simulink model "MenakaModel"  (R2022a)
settings: Solver=ode23tb  StartTime=0.0  StopTime=4  MaxStep=10/(60*24)  RelTol=1e-3
model workspace (MAT data in the model file):
  clima__A_c = 3295.16408265
  clima__A_f = 3100.53942116
  clima__G0 = [0.05; 0.00070738]
  clima__H = 7.9995824611
  clima__T0 = [287.15; 287.15; 287.15; 287.15]
  clima__T_ss = 280.150340169
  clima__alpha_c = 0.0100640347387
  clima__alpha_f = 0.0111385012129
  clima__alpha_i = 0.1
  clima__c_s = [1081 1081]
  clima__cd_c = 8736
  clima__d_c = 1.5
  clima__hour0 = 1
  clima__int_air_speed = 0.5
  clima__l_s = [0.1 0.1]
  clima__lam_s = [2.5 0.85]
  clima__minWindows = 0.299965865643
  clima__rhod_s = [2600 2500]
  clima__tau_c = 1
  crop__A_v = 2080
  crop__C = [0.01 0.001 0.01 0.01]
  crop__C_buf_max = 0.02
  crop__C_wv = 0.2
  crop__Chi_nutrients = [0.015625; 0.0104166666667; 0.00520833333333; 0.00208333333333; 0.00208333333333; 0.00104166666667; 0; 0]
  crop__N = [0; 0; 0; 0; 0; 0; 0; 0]
  crop__R = [0 0 0]
  crop__T_max_v = 40
  crop__T_max_v24 = 27
  crop__T_min_v = 6
  crop__T_min_v24 = 14
  crop__T_sum_end = 1035
  crop__T_v_start_fruit = 1100
  crop__Tsum = 0
  crop__Tv = 288
  crop__b_N_uptake = 0.5
  crop__c_fruit_g = 0.27
  crop__c_fruit_m = 2.3e-07
  crop__c_leaf_g = 0.28
  crop__c_leaf_m = 3.47e-07
  crop__c_stem_g = 0.3
  crop__c_stem_m = 1.47e-07
  crop__fraction_DM = 0.08
  crop__int_air_speed = 0.5
  crop__min_water_capacity = 0.1
  crop__plants_density = 2.1562
  crop__rg_fruit = 2e-07
  crop__rg_leaf = 9.5e-08
  crop__rg_stem = 7.4e-08
  crop__s_buforg_buf = -5000
  crop__s_max_T = 0.5793
  crop__s_max_T24 = 1.3904
  crop__s_min_T = -0.869
  crop__s_min_T24 = -1.1587
  heater__A_e = 0.0001
  heater__A_i = 0.008
  heater__T = 288
  heater__c = 5e-10
  heater__power = 60000000
  screen__Power = 100
  screen__Radthreshold = 900
  screen__beta = 2.23564167038e-14
  screen__gamma_max = 2.26308905438e-14
  screen__velocity = 0.333333333333
  subtrate__C_ws = 0.1
  subtrate__N = [0; 0; 0; 0; 0; 0; 0; 0]
  subtrate__Nmin_subs = 1e-09
  subtrate__Vmax_subs = 10
  subtrate__Vmin_subs = 0.01
  subtrate__sigma_max = 1
  subtrate__sigma_min = 1
  tomato__Cfruit0 = 0.001
  windows__AR = 19.9974923936
  windows__Power = 100
  windows__RadThreshold = 10
  windows__max_night = 10
  windows__tau = 600
undefined symbols (not defined in the file or in its folder): CO2_ppm_ext, Gain_control_Tv_mean, Gain_control_Tv_mean_superior, gain_max_night, GAIN_WIN, Hmax, Hstart, max_night, maxvelocity, RadTh_windows, Radthhold, shift_temp_heat, tau_win, tend_crop1, tend_crop2, tinit_crop1, tinit_crop2, Tmax, Tmax_mean, Tstart, Tven_max, Tven_start, WinAR
libraries: HORTISIM x26, simulink x6
(part 2 of 5)

== system MenakaModel/Control System/Control System Proportional (Ti) + Tmu Windows Relay/Subsystem1 ==
  " " : Inport
  Bus Creator1 : BusCreator  Inputs=2
  Bus Selector : BusSelector  OutputSignals=value,AR
  Rate Limiter : RateLimiter  RisingSlewLimit=maxvelocity*60*24  FallingSlewLimit=-maxvelocity*60*24  SampleTimeMode=inherited
  Out1 : Outport
  wires:
  " "/1 -> Bus Selector/1
  Bus Selector/2 -> Bus Creator1/2  "<AR>"
  Bus Selector/1 -> Rate Limiter/1  "<value>"
  Bus Creator1/1 -> Out1/1
  Rate Limiter/1 -> Bus Creator1/1  "value"

== system MenakaModel/Control System/Control System Proportional (Ti) + Tmu Windows Relay/Windows Controler ==
  note: Subsystem1
  In Bus Element1 : Inport  PortName=IC  Element=Temp.Tair
  In Bus Element2 : Inport  PortName=IC  Element=Gas.HRInt
  Tstart : Inport  Port=2
  Tmax : Inport  Port=3
  Hstart : Inport  Port=4
  Hmax : Inport  Port=5
  R : Inport  Port=6
  Abs : Abs  ZeroCross=off  SaturateOnIntegerOverflow=off
  Bus Creator : BusCreator  Inputs=2
  Bus Selector : BusSelector  OutputSignals=Rad
  Constant : Constant  Value=AR
  Gain : Gain  Gain=100/tau
  Gain1 : Gain  Gain=Power
  Gain2 : Gain  Gain=24*3600*GAIN_WIN
  Integrator : Integrator
  Integrator1 : Integrator  InitialConditionSource=external
  Minus : Sum  Inputs=+-
  Minus1 : Sum  Inputs=+-
  Sec2Days : Gain  Gain=24*3600
  Subsystem : Subsystem
      settings: PortSchema="{\"entries\":[{\"content\":{\"sides\":[{\"content\":{\"connectorIds\":[\"In1\",\"In2\",\"In3\",\"In4\",\"In5\",\"In6\"]},\"type\":\"ConnectorPlacement.EquallySpacedRectSide\",\"uuid\":\"18d05740-181f-409c-94ea-b42b6e57ea74\"},{\"content\":{\"connectorIds\":[\"Out1\"],\"side\":\"RIGHT\"},\"type\":\"ConnectorPlacement.EquallySpacedRectSide\",\"uuid\":\"978406c3-d241-44cd-a3e7-fe734e3a171e\"},{\"content\":{\"connectorIds\":[\"In7\"],\"side\":\"TOP\"},\"type\":\"ConnectorPlacement.EquallySpacedRectSide\",\"uuid\":\"b3c10a0e-c6d9-4444-97f2-9f0c7dea8ec9\"}]},\"type\":\"ConnectorPlacement.EquallySpacedConnector\",\"uuid\":\"429bf3f5-5806-495e-b66b-96810540e6d1\"}],\"packageUris\":[\"http://schema.mathworks.com/mf0/Connector/R2020b\"],\"version\":\"1.0\"}"
  Tanh : Trigonometry  Operator=tanh
  Windows : Outport
  Consumptions : Outport  Port=2
  tag scope: Rad_win=global
  wires:
  Tstart/1 -> Subsystem/1(Tstart)
  In Bus Element1/1 -> Subsystem/2(Ti)
  Tmax/1 -> Subsystem/3(Tmax)
  Integrator/1 -> Bus Creator/1, Minus/2  "value"
  In Bus Element2/1 -> Subsystem/4(HRInt)
  Hstart/1 -> Subsystem/5(HRStart)
  Hmax/1 -> Subsystem/6(HRMax)
  Subsystem/1(y) -> Minus/1
  Sec2Days/1 -> Integrator/1
  Gain1/1 -> Consumptions/1  "Power"
  Abs/1 -> Gain1/1
  Gain/1 -> Abs/1, Sec2Days/1
  Tanh/1 -> Gain/1
  Minus/1 -> Tanh/1
  Bus Creator/1 -> Windows/1
  Constant/1 -> Bus Creator/2  "AR"
  Gain2/1 -> Integrator1/1
  Minus1/1 -> Gain2/1
  Integrator1/1 -> [Rad_win], Subsystem/7(Rad), Minus1/2
  R/1 -> Bus Selector/1
  Bus Selector/1 -> Integrator1/2, Minus1/1  "<Rad>"

== system MenakaModel/Control System/ON//OFF - constant setpoints/Subsystem ==
  Heater : Inport
  C1 : Inport  Port=2
  C2 : Inport  Port=3
  Bus Selector : BusSelector  OutputSignals=HeatVars.QV,HeatVars.QT,A_v,CC
  Bus Selector1 : BusSelector  OutputSignals=HeatVars.QV,HeatVars.QT,CC
  "Scalar2Bus " : Subsystem
  Sum : Sum  Inputs=+++
  Sum1 : Sum  Inputs=++|
  Sum2 : Sum  Inputs=++|
  CoCl : Outport
  wires:
  C1/1 -> Bus Selector/1
  C2/1 -> Bus Selector1/1
  Bus Selector/4 -> Sum2/2  "<CC>"
  Sum/1 -> "Scalar2Bus "/1(QV)
  Sum1/1 -> "Scalar2Bus "/2(QT)
  Bus Selector/1 -> Sum/3  "<QV>"
  Bus Selector1/1 -> Sum/1  "<QV>"
  Bus Selector1/2 -> Sum1/1  "<QT>"
  Bus Selector/3 -> "Scalar2Bus "/3(A)  "<A_v>"
  "Scalar2Bus "/1(CoCl) -> CoCl/1
  Sum2/1 -> "Scalar2Bus "/4(CC)
  Bus Selector1/3 -> Sum2/1  "<CC>"
  Heater/1 -> Sum/2
  Bus Selector/2 -> Sum1/2  "<QT>"

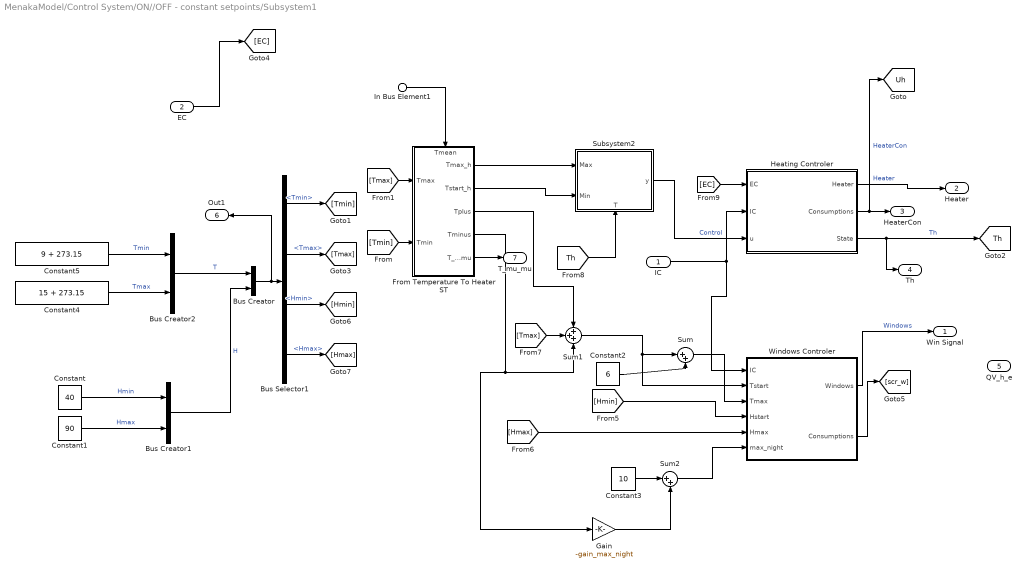
== system MenakaModel/Control System/ON//OFF - constant setpoints/Subsystem1 ==
  IC : Inport
  EC : Inport  Port=2
  In Bus Element1 : Inport  Port=3  PortName=Crop  Element=HeatVars.TvegMean
  Bus Creator : BusCreator  Inputs=2
  Bus Creator1 : BusCreator  Inputs=2
  Bus Creator2 : BusCreator  Inputs=2
  Bus Selector1 : BusSelector  OutputSignals=T.Tmin,T.Tmax,H.Hmin,H.Hmax
  Constant : Constant  Value=40
  Constant1 : Constant  Value=90
  Constant2 : Constant  Value=6
  Constant3 : Constant  Value=10
  Constant4 : Constant  Value=15 + 273.15
  Constant5 : Constant  Value=9 + 273.15
  From Temperature To Heater ST : Subsystem
      settings: PortSchema="{\"entries\":[{\"content\":{\"sides\":[{\"content\":{\"connectorIds\":[\"In1\",\"In2\"]},\"type\":\"ConnectorPlacement.EquallySpacedRectSide\",\"uuid\":\"89e621f6-ef56-4bf6-8223-627da8dff273\"},{\"content\":{\"connectorIds\":[\"Out1\",\"Out2\",\"Out3\",\"Out4\",\"Out5\"],\"side\":\"RIGHT\"},\"type\":\"ConnectorPlacement.EquallySpacedRectSide\",\"uuid\":\"65a656ef-c181-4216-a438-20c957365b5a\"},{\"content\":{\"connectorIds\":[\"In3\"],\"side\":\"TOP\"},\"type\":\"ConnectorPlacement.EquallySpacedRectSide\",\"uuid\":\"92fb86b4-e089-4bcc-a83f-ddbdae4e02ae\"}]},\"type\":\"ConnectorPlacement.EquallySpacedConnector\",\"uuid\":\"5ba309fb-c1b1-411e-b7b8-8afa0be10efe\"}],\"packageUris\":[\"http://schema.mathworks.com/mf0/Connector/R2020b\"],\"version\":\"1.0\"}"
  Gain : Gain  Gain=-gain_max_night
  Heating Controler : Subsystem  AncestorBlock=HORTISIM/Climate/Controls/Heating Controler  mask{T=288, power=1000e3, A_e=6e-4, A_i=6e-4, c=1e-8}
      mask DialogControl InitialCondition Prompt: Initial Condition
      mask DialogControl Parameters Prompt: Parameters
      mask Display: image('$imagefile'); % Use "Edit Image" on toolstrip to change.
  Subsystem2 : Subsystem
      settings: PortSchema="{\"entries\":[{\"content\":{\"sides\":[{\"content\":{\"connectorIds\":[\"In1\",\"In2\"]},\"type\":\"ConnectorPlacement.EquallySpacedRectSide\",\"uuid\":\"063c50bb-990a-4f1b-9201-b176301531ab\"},{\"content\":{\"connectorIds\":[\"Out1\"],\"side\":\"RIGHT\"},\"type\":\"ConnectorPlacement.EquallySpacedRectSide\",\"uuid\":\"3a0e99c4-d22b-4375-8de8-a1d36b289de2\"},{\"content\":{\"connectorIds\":[],\"side\":\"TOP\"},\"type\":\"ConnectorPlacement.EquallySpacedRectSide\",\"uuid\":\"03cb5fb9-820c-4863-975f-3967583da0d3\"},{\"content\":{\"connectorIds\":[\"In3\"],\"side\":\"BOTTOM\"},\"type\":\"ConnectorPlacement.EquallySpacedRectSide\",\"uuid\":\"69ae3c50-5771-48e7-9488-918c6831cfd5\"}]},\"type\":\"ConnectorPlacement.EquallySpacedConnector\",\"uuid\":\"dc439741-a5d5-4759-903e-5ad1ebb8fa8a\"}],\"packageUris\":[\"http://schema.mathworks.com/mf0/Connector/R2020b\"],\"version\":\"1.0\"}"
  Sum : Sum  Inputs=|++
  Sum1 : Sum  Inputs=+++
  Sum2 : Sum  Inputs=|++
  Windows Controler : Subsystem  AncestorBlock=HORTISIM/Climate/Controls/Windows Controler  mask{Power=100, max_night=10, tau=tau_win, RadThreshold=100, AR=10}
      mask Display: image('$imagefile'); % Use "Edit Image" on toolstrip to change.
  Win Signal : Outport
  Heater : Outport  Port=2
  HeaterCon : Outport  Port=3
  Th : Outport  Port=4
  QV_h_e : Outport  Port=5
  Out1 : Outport  Port=6
  T_mu_mu : Outport  Port=7
  tag scope: Th=global, Uh=global
  wires:
  From Temperature To Heater ST/1(Tmax_h) -> Subsystem2/1(Max)
  Bus Creator2/1 -> Bus Creator/1  "T"
  Sum/1 -> Windows Controler/3(Tmax)
  EC/1 -> [EC]
  Bus Selector1/4 -> [Hmax]  "<Hmax>"
  Constant1/1 -> Bus Creator1/2  "Hmax"
  Constant5/1 -> Bus Creator2/1  "Tmin"
  Bus Selector1/3 -> [Hmin]  "<Hmin>"
  Bus Creator/1 -> Out1/1, Bus Selector1/1
  Windows Controler/1(Windows) -> Win Signal/1  "Windows"
  [Tmin] -> From Temperature To Heater ST/2(Tmin)
  Heating Controler/1(Heater) -> Heater/1  "Heater"
  Constant2/1 -> Sum/2
  [Tmax] -> From Temperature To Heater ST/1(Tmax)
  Heating Controler/2(Consumptions) -> HeaterCon/1, [Uh]  "HeaterCon"
  Constant4/1 -> Bus Creator2/2  "Tmax"
  Constant/1 -> Bus Creator1/1  "Hmin"
  Bus Selector1/1 -> [Tmin]  "<Tmin>"
  Heating Controler/3(State) -> Th/1, [Th]  "Th"
  [Hmax] -> Windows Controler/5(Hmax)
  [EC] -> Heating Controler/1(EC)
  [Hmin] -> Windows Controler/4(Hstart)
  Subsystem2/1(y) -> Heating Controler/3(u)  "Control"
  [Th] -> Subsystem2/3(T)
  Windows Controler/2(Consumptions) -> [scr_w]
  Sum1/1 -> Sum/1, Windows Controler/2(Tstart)
  Bus Creator1/1 -> Bus Creator/2  "H"
  Bus Selector1/2 -> [Tmax]  "<Tmax>"
  From Temperature To Heater ST/2(Tstart_h) -> Subsystem2/2(" Min")
  In Bus Element1/1 -> From Temperature To Heater ST/3(Tmean)
  [Tmax] -> Sum1/2
  From Temperature To Heater ST/3(Tplus) -> Sum1/1
  From Temperature To Heater ST/4(Tminus) -> Sum1/3, Gain/1
  Constant3/1 -> Sum2/1
  Sum2/1 -> Windows Controler/6(max_night)
  Gain/1 -> Sum2/2
  From Temperature To Heater ST/5(T_mu_mu) -> T_mu_mu/1
  IC/1 -> Heating Controler/2(IC), Windows Controler/1(IC)

== system MenakaModel/Control System/PID - const st - Ti mesure - Dynamics ST/Subsystem ==
  Heater : Inport
  C1 : Inport  Port=2
  C2 : Inport  Port=3
  Bus Selector : BusSelector  OutputSignals=HeatVars.QV,HeatVars.QT,A_v,CC
  Bus Selector1 : BusSelector  OutputSignals=HeatVars.QV,HeatVars.QT,CC
  "Scalar2Bus " : Subsystem
  Sum : Sum  Inputs=+++
  Sum1 : Sum  Inputs=++|
  Sum2 : Sum  Inputs=++|
  CoCl : Outport
  wires:
  C1/1 -> Bus Selector/1
  C2/1 -> Bus Selector1/1
  Bus Selector/4 -> Sum2/2  "<CC>"
  Sum/1 -> "Scalar2Bus "/1(QV)
  Sum1/1 -> "Scalar2Bus "/2(QT)
  Bus Selector/1 -> Sum/3  "<QV>"
  Bus Selector1/1 -> Sum/1  "<QV>"
  Bus Selector1/2 -> Sum1/1  "<QT>"
  Bus Selector/3 -> "Scalar2Bus "/3(A)  "<A_v>"
  "Scalar2Bus "/1(CoCl) -> CoCl/1
  Sum2/1 -> "Scalar2Bus "/4(CC)
  Bus Selector1/3 -> Sum2/1  "<CC>"
  Heater/1 -> Sum/2
  Bus Selector/2 -> Sum1/2  "<QT>"

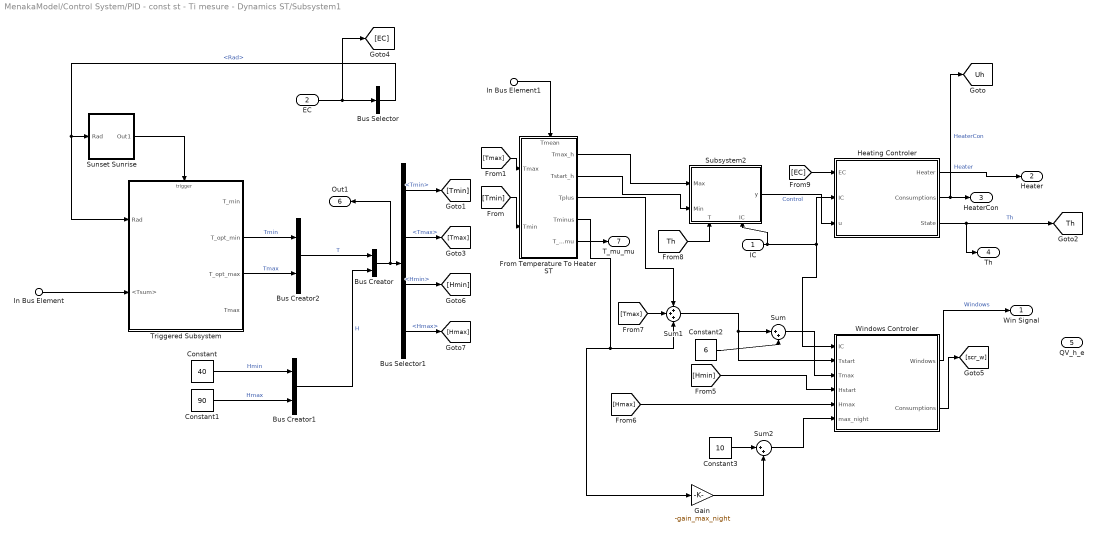
== system MenakaModel/Control System/PID - const st - Ti mesure - Dynamics ST/Subsystem1 ==
  IC : Inport
  EC : Inport  Port=2
  In Bus Element : Inport  Port=3  PortName=Crop  Element=Tsum
  In Bus Element1 : Inport  Port=3  PortName=Crop  Element=HeatVars.TvegMean
  Bus Creator : BusCreator  Inputs=2
  Bus Creator1 : BusCreator  Inputs=2
  Bus Creator2 : BusCreator  Inputs=2
  Bus Selector : BusSelector  OutputSignals=Rad
  Bus Selector1 : BusSelector  OutputSignals=T.Tmin,T.Tmax,H.Hmin,H.Hmax
  Constant : Constant  Value=40
  Constant1 : Constant  Value=90
  Constant2 : Constant  Value=6
  Constant3 : Constant  Value=10
  From Temperature To Heater ST : Subsystem
      settings: PortSchema="{\"entries\":[{\"content\":{\"sides\":[{\"content\":{\"connectorIds\":[\"In1\",\"In2\"]},\"type\":\"ConnectorPlacement.EquallySpacedRectSide\",\"uuid\":\"8e56c99b-44f6-44c1-b47c-48add3c8a511\"},{\"content\":{\"connectorIds\":[\"Out1\",\"Out2\",\"Out3\",\"Out4\",\"Out5\"],\"side\":\"RIGHT\"},\"type\":\"ConnectorPlacement.EquallySpacedRectSide\",\"uuid\":\"935a66df-2dd1-4f44-b4bf-88934f25c0cb\"},{\"content\":{\"connectorIds\":[\"In3\"],\"side\":\"TOP\"},\"type\":\"ConnectorPlacement.EquallySpacedRectSide\",\"uuid\":\"2b3b0ca2-0cfb-4129-af85-fa3b6a689c74\"}]},\"type\":\"ConnectorPlacement.EquallySpacedConnector\",\"uuid\":\"4599665f-2afd-48c1-b4f2-02758b438fe7\"}],\"packageUris\":[\"http://schema.mathworks.com/mf0/Connector/R2020b\"],\"version\":\"1.0\"}"
  Gain : Gain  Gain=-gain_max_night
  Heating Controler : Subsystem  AncestorBlock=HORTISIM/Climate/Controls/Heating Controler  mask{T=288, power=1000e3, A_e=6e-4, A_i=6e-4, c=1e-8}
      mask DialogControl InitialCondition Prompt: Initial Condition
      mask DialogControl Parameters Prompt: Parameters
      mask Display: image('$imagefile'); % Use "Edit Image" on toolstrip to change.
  Subsystem2 : Subsystem  Variant=on  VariantControlMode=label  VariantControl=Choice  LabelModeActiveChoice=Choice_1
      settings: PortSchema="{\"entries\":[{\"content\":{\"sides\":[{\"content\":{\"connectorIds\":[\"In1\",\"In2\"]},\"type\":\"ConnectorPlacement.EquallySpacedRectSide\",\"uuid\":\"76a0539e-cd8b-47df-82d9-61971d3be914\"},{\"content\":{\"connectorIds\":[\"Out1\"],\"side\":\"RIGHT\"},\"type\":\"ConnectorPlacement.EquallySpacedRectSide\",\"uuid\":\"93f2ebb7-6ab4-4fcc-bc7a-3583f1db6e8e\"},{\"content\":{\"connectorIds\":[],\"side\":\"TOP\"},\"type\":\"ConnectorPlacement.EquallySpacedRectSide\",\"uuid\":\"b50a0ff6-3876-4dcb-8bb9-79340929aa80\"},{\"content\":{\"connectorIds\":[\"In3\",\"In4\"],\"side\":\"BOTTOM\"},\"type\":\"ConnectorPlacement.EquallySpacedRectSide\",\"uuid\":\"63f2a7a5-83ef-48e2-af90-7d61b47411e6\"}]},\"type\":\"ConnectorPlacement.EquallySpacedConnector\",\"uuid\":\"d97900b9-3143-4b55-b66d-f73dd0302926\"}],\"packageUris\":[\"http://schema.mathworks.com/mf0/Connector/R2020b\"],\"version\":\"1.0\"}"
  Sum : Sum  Inputs=|++
  Sum1 : Sum  Inputs=+++
  Sum2 : Sum  Inputs=|++
  Sunset Sunrise : Subsystem
  Triggered Subsystem : Subsystem  TreatAsAtomicUnit=on
  Windows Controler : Subsystem  AncestorBlock=HORTISIM/Climate/Controls/Windows Controler  mask{Power=100, max_night=10, tau=tau_win, RadThreshold=100, AR=10}
      mask Display: image('$imagefile'); % Use "Edit Image" on toolstrip to change.
  Win Signal : Outport
  Heater : Outport  Port=2
  HeaterCon : Outport  Port=3
  Th : Outport  Port=4
  QV_h_e : Outport  Port=5
  Out1 : Outport  Port=6
  T_mu_mu : Outport  Port=7
  tag scope: Th=global, Uh=global
  wires:
  Bus Selector/1 -> Triggered Subsystem/1(Rad), Sunset Sunrise/1(Rad)  "<Rad>"
  Bus Creator2/1 -> Bus Creator/1  "T"
  Sunset Sunrise/1(Out1) -> Triggered Subsystem/Trigger
  Sum/1 -> Windows Controler/3(Tmax)
  EC/1 -> [EC], Bus Selector/1
  Bus Selector1/4 -> [Hmax]  "<Hmax>"
  Constant1/1 -> Bus Creator1/2  "Hmax"
  Triggered Subsystem/2(T_opt_min) -> Bus Creator2/1  "Tmin"
  Bus Selector1/3 -> [Hmin]  "<Hmin>"
  Bus Creator/1 -> Out1/1, Bus Selector1/1
  Windows Controler/1(Windows) -> Win Signal/1  "Windows"
  [Tmin] -> From Temperature To Heater ST/2(Tmin)
  In Bus Element/1 -> Triggered Subsystem/2(<Tsum>)
  Heating Controler/1(Heater) -> Heater/1  "Heater"
  Constant2/1 -> Sum/2
  [Tmax] -> From Temperature To Heater ST/1(Tmax)
  Heating Controler/2(Consumptions) -> HeaterCon/1, [Uh]  "HeaterCon"
  Triggered Subsystem/3(T_opt_max) -> Bus Creator2/2  "Tmax"
  Constant/1 -> Bus Creator1/1  "Hmin"
  Bus Selector1/1 -> [Tmin]  "<Tmin>"
  Heating Controler/3(State) -> Th/1, [Th]  "Th"
  [Hmax] -> Windows Controler/5(Hmax)
  [EC] -> Heating Controler/1(EC)
  [Hmin] -> Windows Controler/4(Hstart)
  Windows Controler/2(Consumptions) -> [scr_w]
  Sum1/1 -> Sum/1, Windows Controler/2(Tstart)
  Bus Creator1/1 -> Bus Creator/2  "H"
  Bus Selector1/2 -> [Tmax]  "<Tmax>"
  In Bus Element1/1 -> From Temperature To Heater ST/3(Tmean)
  [Tmax] -> Sum1/2
  From Temperature To Heater ST/3(Tplus) -> Sum1/1
  From Temperature To Heater ST/4(Tminus) -> Sum1/3, Gain/1
  Constant3/1 -> Sum2/1
  Sum2/1 -> Windows Controler/6(max_night)
  Gain/1 -> Sum2/2
  From Temperature To Heater ST/5(T_mu_mu) -> T_mu_mu/1
  IC/1 -> Heating Controler/2(IC), Windows Controler/1(IC), Subsystem2/4(IC)
  From Temperature To Heater ST/1(Tmax_h) -> Subsystem2/1(Max)
  From Temperature To Heater ST/2(Tstart_h) -> Subsystem2/2(" Min")
  [Th] -> Subsystem2/3(T)
  Subsystem2/1(y) -> Heating Controler/3(u)  "Control"

== system MenakaModel/Control System/PID - constant setpoints/Subsystem ==
  Heater : Inport
  C1 : Inport  Port=2
  C2 : Inport  Port=3
  Bus Selector : BusSelector  OutputSignals=HeatVars.QV,HeatVars.QT,A_v,CC
  Bus Selector1 : BusSelector  OutputSignals=HeatVars.QV,HeatVars.QT,CC
  "Scalar2Bus " : Subsystem
  Sum : Sum  Inputs=+++
  Sum1 : Sum  Inputs=++|
  Sum2 : Sum  Inputs=++|
  CoCl : Outport
  wires:
  C1/1 -> Bus Selector/1
  C2/1 -> Bus Selector1/1
  Bus Selector/4 -> Sum2/2  "<CC>"
  Sum/1 -> "Scalar2Bus "/1(QV)
  Sum1/1 -> "Scalar2Bus "/2(QT)
  Bus Selector/1 -> Sum/3  "<QV>"
  Bus Selector1/1 -> Sum/1  "<QV>"
  Bus Selector1/2 -> Sum1/1  "<QT>"
  Bus Selector/3 -> "Scalar2Bus "/3(A)  "<A_v>"
  "Scalar2Bus "/1(CoCl) -> CoCl/1
  Sum2/1 -> "Scalar2Bus "/4(CC)
  Bus Selector1/3 -> Sum2/1  "<CC>"
  Heater/1 -> Sum/2
  Bus Selector/2 -> Sum1/2  "<QT>"

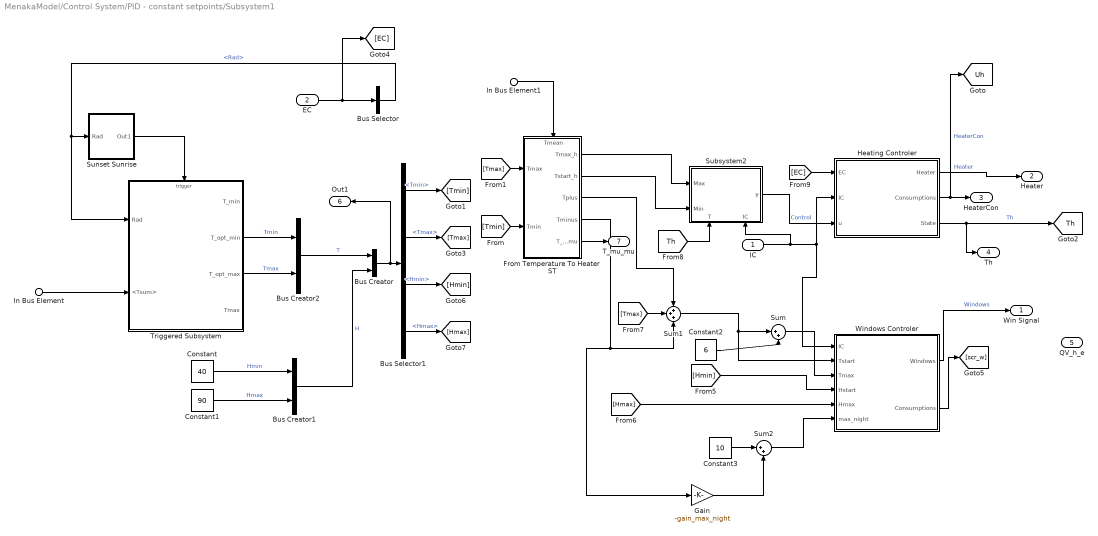
== system MenakaModel/Control System/PID - constant setpoints/Subsystem1 ==
  IC : Inport
  EC : Inport  Port=2
  In Bus Element : Inport  Port=3  PortName=Crop  Element=Tsum
  In Bus Element1 : Inport  Port=3  PortName=Crop  Element=HeatVars.TvegMean
  Bus Creator : BusCreator  Inputs=2
  Bus Creator1 : BusCreator  Inputs=2
  Bus Creator2 : BusCreator  Inputs=2
  Bus Selector : BusSelector  OutputSignals=Rad
  Bus Selector1 : BusSelector  OutputSignals=T.Tmin,T.Tmax,H.Hmin,H.Hmax
  Constant : Constant  Value=40
  Constant1 : Constant  Value=90
  Constant2 : Constant  Value=6
  Constant3 : Constant  Value=10
  From Temperature To Heater ST : Subsystem
      settings: PortSchema="{\"entries\":[{\"content\":{\"sides\":[{\"content\":{\"connectorIds\":[\"In1\",\"In2\"]},\"type\":\"ConnectorPlacement.EquallySpacedRectSide\",\"uuid\":\"89e621f6-ef56-4bf6-8223-627da8dff273\"},{\"content\":{\"connectorIds\":[\"Out1\",\"Out2\",\"Out3\",\"Out4\",\"Out5\"],\"side\":\"RIGHT\"},\"type\":\"ConnectorPlacement.EquallySpacedRectSide\",\"uuid\":\"65a656ef-c181-4216-a438-20c957365b5a\"},{\"content\":{\"connectorIds\":[\"In3\"],\"side\":\"TOP\"},\"type\":\"ConnectorPlacement.EquallySpacedRectSide\",\"uuid\":\"92fb86b4-e089-4bcc-a83f-ddbdae4e02ae\"}]},\"type\":\"ConnectorPlacement.EquallySpacedConnector\",\"uuid\":\"5ba309fb-c1b1-411e-b7b8-8afa0be10efe\"}],\"packageUris\":[\"http://schema.mathworks.com/mf0/Connector/R2020b\"],\"version\":\"1.0\"}"
  Gain : Gain  Gain=-gain_max_night
  Heating Controler : Subsystem  AncestorBlock=HORTISIM/Climate/Controls/Heating Controler  mask{T=288, power=1000e3, A_e=6e-4, A_i=6e-4, c=1e-8}
      mask DialogControl InitialCondition Prompt: Initial Condition
      mask DialogControl Parameters Prompt: Parameters
      mask Display: image('$imagefile'); % Use "Edit Image" on toolstrip to change.
  Subsystem2 : Subsystem
      settings: PortSchema="{\"entries\":[{\"content\":{\"sides\":[{\"content\":{\"connectorIds\":[\"In1\",\"In2\"]},\"type\":\"ConnectorPlacement.EquallySpacedRectSide\",\"uuid\":\"76a0539e-cd8b-47df-82d9-61971d3be914\"},{\"content\":{\"connectorIds\":[\"Out1\"],\"side\":\"RIGHT\"},\"type\":\"ConnectorPlacement.EquallySpacedRectSide\",\"uuid\":\"93f2ebb7-6ab4-4fcc-bc7a-3583f1db6e8e\"},{\"content\":{\"connectorIds\":[],\"side\":\"TOP\"},\"type\":\"ConnectorPlacement.EquallySpacedRectSide\",\"uuid\":\"b50a0ff6-3876-4dcb-8bb9-79340929aa80\"},{\"content\":{\"connectorIds\":[\"In3\",\"In4\"],\"side\":\"BOTTOM\"},\"type\":\"ConnectorPlacement.EquallySpacedRectSide\",\"uuid\":\"63f2a7a5-83ef-48e2-af90-7d61b47411e6\"}]},\"type\":\"ConnectorPlacement.EquallySpacedConnector\",\"uuid\":\"d97900b9-3143-4b55-b66d-f73dd0302926\"}],\"packageUris\":[\"http://schema.mathworks.com/mf0/Connector/R2020b\"],\"version\":\"1.0\"}"
  Sum : Sum  Inputs=|++
  Sum1 : Sum  Inputs=+++
  Sum2 : Sum  Inputs=|++
  Sunset Sunrise : Subsystem
  Triggered Subsystem : Subsystem  TreatAsAtomicUnit=on
  Windows Controler : Subsystem  AncestorBlock=HORTISIM/Climate/Controls/Windows Controler  mask{Power=100, max_night=10, tau=tau_win, RadThreshold=100, AR=10}
      mask Display: image('$imagefile'); % Use "Edit Image" on toolstrip to change.
  Win Signal : Outport
  Heater : Outport  Port=2
  HeaterCon : Outport  Port=3
  Th : Outport  Port=4
  QV_h_e : Outport  Port=5
  Out1 : Outport  Port=6
  T_mu_mu : Outport  Port=7
  tag scope: Th=global, Uh=global
  wires:
  Bus Selector/1 -> Triggered Subsystem/1(Rad), Sunset Sunrise/1(Rad)  "<Rad>"
  From Temperature To Heater ST/1(Tmax_h) -> Subsystem2/1(Max)
  Bus Creator2/1 -> Bus Creator/1  "T"
  Sunset Sunrise/1(Out1) -> Triggered Subsystem/Trigger
  Sum/1 -> Windows Controler/3(Tmax)
  EC/1 -> [EC], Bus Selector/1
  Bus Selector1/4 -> [Hmax]  "<Hmax>"
  Constant1/1 -> Bus Creator1/2  "Hmax"
  Triggered Subsystem/2(T_opt_min) -> Bus Creator2/1  "Tmin"
  Bus Selector1/3 -> [Hmin]  "<Hmin>"
  Bus Creator/1 -> Out1/1, Bus Selector1/1
  Windows Controler/1(Windows) -> Win Signal/1  "Windows"
  [Tmin] -> From Temperature To Heater ST/2(Tmin)
  In Bus Element/1 -> Triggered Subsystem/2(<Tsum>)
  Heating Controler/1(Heater) -> Heater/1  "Heater"
  Constant2/1 -> Sum/2
  [Tmax] -> From Temperature To Heater ST/1(Tmax)
  Heating Controler/2(Consumptions) -> HeaterCon/1, [Uh]  "HeaterCon"
  Triggered Subsystem/3(T_opt_max) -> Bus Creator2/2  "Tmax"
  Constant/1 -> Bus Creator1/1  "Hmin"
  Bus Selector1/1 -> [Tmin]  "<Tmin>"
  Heating Controler/3(State) -> Th/1, [Th]  "Th"
  [Hmax] -> Windows Controler/5(Hmax)
  [EC] -> Heating Controler/1(EC)
  [Hmin] -> Windows Controler/4(Hstart)
  Subsystem2/1(y) -> Heating Controler/3(u)  "Control"
  [Th] -> Subsystem2/3(T)
  Windows Controler/2(Consumptions) -> [scr_w]
  Sum1/1 -> Sum/1, Windows Controler/2(Tstart)
  Bus Creator1/1 -> Bus Creator/2  "H"
  Bus Selector1/2 -> [Tmax]  "<Tmax>"
  From Temperature To Heater ST/2(Tstart_h) -> Subsystem2/2(" Min")
  In Bus Element1/1 -> From Temperature To Heater ST/3(Tmean)
  [Tmax] -> Sum1/2
  From Temperature To Heater ST/3(Tplus) -> Sum1/1
  From Temperature To Heater ST/4(Tminus) -> Sum1/3, Gain/1
  Constant3/1 -> Sum2/1
  Sum2/1 -> Windows Controler/6(max_night)
  Gain/1 -> Sum2/2
  From Temperature To Heater ST/5(T_mu_mu) -> T_mu_mu/1
  IC/1 -> Subsystem2/4(IC), Heating Controler/2(IC), Windows Controler/1(IC)

== system MenakaModel/Control System/PID - constant setpoints - Ti measure/Subsystem ==
  Heater : Inport
  C1 : Inport  Port=2
  C2 : Inport  Port=3
  Bus Selector : BusSelector  OutputSignals=HeatVars.QV,HeatVars.QT,A_v,CC
  Bus Selector1 : BusSelector  OutputSignals=HeatVars.QV,HeatVars.QT,CC
  "Scalar2Bus " : Subsystem
  Sum : Sum  Inputs=+++
  Sum1 : Sum  Inputs=++|
  Sum2 : Sum  Inputs=++|
  CoCl : Outport
  wires:
  C1/1 -> Bus Selector/1
  C2/1 -> Bus Selector1/1
  Bus Selector/4 -> Sum2/2  "<CC>"
  Sum/1 -> "Scalar2Bus "/1(QV)
  Sum1/1 -> "Scalar2Bus "/2(QT)
  Bus Selector/1 -> Sum/3  "<QV>"
  Bus Selector1/1 -> Sum/1  "<QV>"
  Bus Selector1/2 -> Sum1/1  "<QT>"
  Bus Selector/3 -> "Scalar2Bus "/3(A)  "<A_v>"
  "Scalar2Bus "/1(CoCl) -> CoCl/1
  Sum2/1 -> "Scalar2Bus "/4(CC)
  Bus Selector1/3 -> Sum2/1  "<CC>"
  Heater/1 -> Sum/2
  Bus Selector/2 -> Sum1/2  "<QT>"

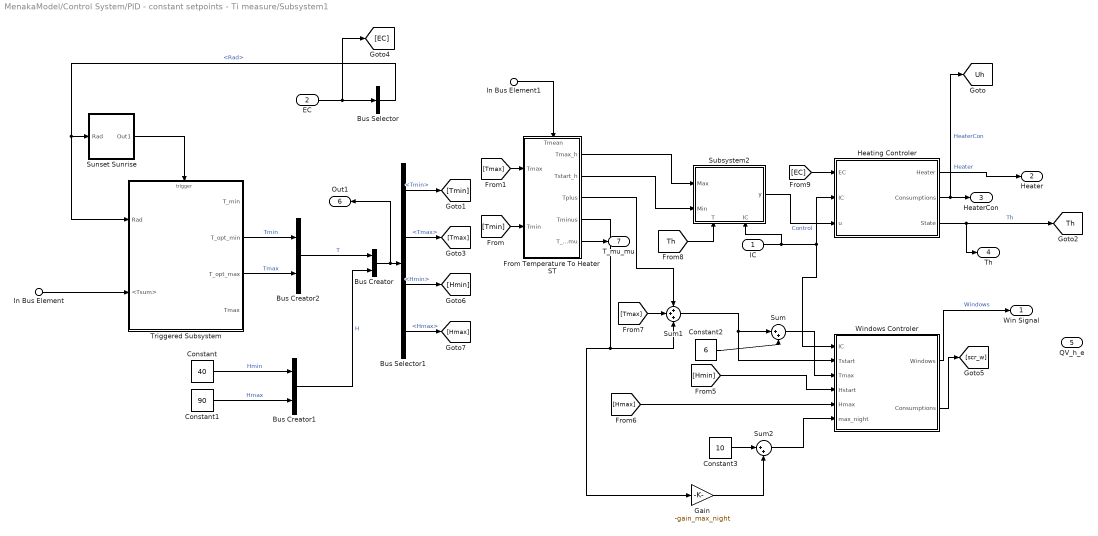
== system MenakaModel/Control System/PID - constant setpoints - Ti measure/Subsystem1 ==
  IC : Inport
  EC : Inport  Port=2
  In Bus Element : Inport  Port=3  PortName=Crop  Element=Tsum
  In Bus Element1 : Inport  Port=3  PortName=Crop  Element=HeatVars.TvegMean
  Bus Creator : BusCreator  Inputs=2
  Bus Creator1 : BusCreator  Inputs=2
  Bus Creator2 : BusCreator  Inputs=2
  Bus Selector : BusSelector  OutputSignals=Rad
  Bus Selector1 : BusSelector  OutputSignals=T.Tmin,T.Tmax,H.Hmin,H.Hmax
  Constant : Constant  Value=40
  Constant1 : Constant  Value=90
  Constant2 : Constant  Value=6
  Constant3 : Constant  Value=10
  From Temperature To Heater ST : Subsystem
      settings: PortSchema="{\"entries\":[{\"content\":{\"sides\":[{\"content\":{\"connectorIds\":[\"In1\",\"In2\"]},\"type\":\"ConnectorPlacement.EquallySpacedRectSide\",\"uuid\":\"89e621f6-ef56-4bf6-8223-627da8dff273\"},{\"content\":{\"connectorIds\":[\"Out1\",\"Out2\",\"Out3\",\"Out4\",\"Out5\"],\"side\":\"RIGHT\"},\"type\":\"ConnectorPlacement.EquallySpacedRectSide\",\"uuid\":\"65a656ef-c181-4216-a438-20c957365b5a\"},{\"content\":{\"connectorIds\":[\"In3\"],\"side\":\"TOP\"},\"type\":\"ConnectorPlacement.EquallySpacedRectSide\",\"uuid\":\"92fb86b4-e089-4bcc-a83f-ddbdae4e02ae\"}]},\"type\":\"ConnectorPlacement.EquallySpacedConnector\",\"uuid\":\"5ba309fb-c1b1-411e-b7b8-8afa0be10efe\"}],\"packageUris\":[\"http://schema.mathworks.com/mf0/Connector/R2020b\"],\"version\":\"1.0\"}"
  Gain : Gain  Gain=-gain_max_night
  Heating Controler : Subsystem  AncestorBlock=HORTISIM/Climate/Controls/Heating Controler  mask{T=288, power=1000e3, A_e=6e-4, A_i=6e-4, c=1e-8}
      mask DialogControl InitialCondition Prompt: Initial Condition
      mask DialogControl Parameters Prompt: Parameters
      mask Display: image('$imagefile'); % Use "Edit Image" on toolstrip to change.
  Subsystem2 : Subsystem  Variant=on  VariantControlMode=label  VariantControl=Choice  LabelModeActiveChoice=Choice_1
      settings: PortSchema="{\"entries\":[{\"content\":{\"sides\":[{\"content\":{\"connectorIds\":[\"In1\",\"In2\"]},\"type\":\"ConnectorPlacement.EquallySpacedRectSide\",\"uuid\":\"76a0539e-cd8b-47df-82d9-61971d3be914\"},{\"content\":{\"connectorIds\":[\"Out1\"],\"side\":\"RIGHT\"},\"type\":\"ConnectorPlacement.EquallySpacedRectSide\",\"uuid\":\"93f2ebb7-6ab4-4fcc-bc7a-3583f1db6e8e\"},{\"content\":{\"connectorIds\":[],\"side\":\"TOP\"},\"type\":\"ConnectorPlacement.EquallySpacedRectSide\",\"uuid\":\"b50a0ff6-3876-4dcb-8bb9-79340929aa80\"},{\"content\":{\"connectorIds\":[\"In3\",\"In4\"],\"side\":\"BOTTOM\"},\"type\":\"ConnectorPlacement.EquallySpacedRectSide\",\"uuid\":\"63f2a7a5-83ef-48e2-af90-7d61b47411e6\"}]},\"type\":\"ConnectorPlacement.EquallySpacedConnector\",\"uuid\":\"d97900b9-3143-4b55-b66d-f73dd0302926\"}],\"packageUris\":[\"http://schema.mathworks.com/mf0/Connector/R2020b\"],\"version\":\"1.0\"}"
  Sum : Sum  Inputs=|++
  Sum1 : Sum  Inputs=+++
  Sum2 : Sum  Inputs=|++
  Sunset Sunrise : Subsystem
  Triggered Subsystem : Subsystem  TreatAsAtomicUnit=on
  Windows Controler : Subsystem  AncestorBlock=HORTISIM/Climate/Controls/Windows Controler  mask{Power=100, max_night=10, tau=tau_win, RadThreshold=100, AR=10}
      mask Display: image('$imagefile'); % Use "Edit Image" on toolstrip to change.
  Win Signal : Outport
  Heater : Outport  Port=2
  HeaterCon : Outport  Port=3
  Th : Outport  Port=4
  QV_h_e : Outport  Port=5
  Out1 : Outport  Port=6
  T_mu_mu : Outport  Port=7
  tag scope: Th=global, Uh=global
  wires:
  Bus Selector/1 -> Triggered Subsystem/1(Rad), Sunset Sunrise/1(Rad)  "<Rad>"
  From Temperature To Heater ST/1(Tmax_h) -> Subsystem2/1(Max)
  Bus Creator2/1 -> Bus Creator/1  "T"
  Sunset Sunrise/1(Out1) -> Triggered Subsystem/Trigger
  Sum/1 -> Windows Controler/3(Tmax)
  EC/1 -> [EC], Bus Selector/1
  Bus Selector1/4 -> [Hmax]  "<Hmax>"
  Constant1/1 -> Bus Creator1/2  "Hmax"
  Triggered Subsystem/2(T_opt_min) -> Bus Creator2/1  "Tmin"
  Bus Selector1/3 -> [Hmin]  "<Hmin>"
  Bus Creator/1 -> Out1/1, Bus Selector1/1
  Windows Controler/1(Windows) -> Win Signal/1  "Windows"
  [Tmin] -> From Temperature To Heater ST/2(Tmin)
  In Bus Element/1 -> Triggered Subsystem/2(<Tsum>)
  Heating Controler/1(Heater) -> Heater/1  "Heater"
  Constant2/1 -> Sum/2
  [Tmax] -> From Temperature To Heater ST/1(Tmax)
  Heating Controler/2(Consumptions) -> HeaterCon/1, [Uh]  "HeaterCon"
  Triggered Subsystem/3(T_opt_max) -> Bus Creator2/2  "Tmax"
  Constant/1 -> Bus Creator1/1  "Hmin"
  Bus Selector1/1 -> [Tmin]  "<Tmin>"
  Heating Controler/3(State) -> Th/1, [Th]  "Th"
  [Hmax] -> Windows Controler/5(Hmax)
  [EC] -> Heating Controler/1(EC)
  [Hmin] -> Windows Controler/4(Hstart)
  Subsystem2/1(y) -> Heating Controler/3(u)  "Control"
  [Th] -> Subsystem2/3(T)
  Windows Controler/2(Consumptions) -> [scr_w]
  Sum1/1 -> Sum/1, Windows Controler/2(Tstart)
  Bus Creator1/1 -> Bus Creator/2  "H"
  Bus Selector1/2 -> [Tmax]  "<Tmax>"
  From Temperature To Heater ST/2(Tstart_h) -> Subsystem2/2(" Min")
  In Bus Element1/1 -> From Temperature To Heater ST/3(Tmean)
  [Tmax] -> Sum1/2
  From Temperature To Heater ST/3(Tplus) -> Sum1/1
  From Temperature To Heater ST/4(Tminus) -> Sum1/3, Gain/1
  Constant3/1 -> Sum2/1
  Sum2/1 -> Windows Controler/6(max_night)
  Gain/1 -> Sum2/2
  From Temperature To Heater ST/5(T_mu_mu) -> T_mu_mu/1
  IC/1 -> Heating Controler/2(IC), Windows Controler/1(IC), Subsystem2/4(IC)

== system MenakaModel/Control System/PID-set-points/Subsystem ==
  Heater : Inport
  C1 : Inport  Port=2
  C2 : Inport  Port=3
  Bus Selector : BusSelector  OutputSignals=HeatVars.QV,HeatVars.QT,A_v,CC
  Bus Selector1 : BusSelector  OutputSignals=HeatVars.QV,HeatVars.QT,CC
  "Scalar2Bus " : Subsystem
  Sum : Sum  Inputs=+++
  Sum1 : Sum  Inputs=++|
  Sum2 : Sum  Inputs=++|
  CoCl : Outport
  wires:
  C1/1 -> Bus Selector/1
  C2/1 -> Bus Selector1/1
  Bus Selector/4 -> Sum2/2  "<CC>"
  Sum/1 -> "Scalar2Bus "/1(QV)
  Sum1/1 -> "Scalar2Bus "/2(QT)
  Bus Selector/1 -> Sum/3  "<QV>"
  Bus Selector1/1 -> Sum/1  "<QV>"
  Bus Selector1/2 -> Sum1/1  "<QT>"
  Bus Selector/3 -> "Scalar2Bus "/3(A)  "<A_v>"
  "Scalar2Bus "/1(CoCl) -> CoCl/1
  Sum2/1 -> "Scalar2Bus "/4(CC)
  Bus Selector1/3 -> Sum2/1  "<CC>"
  Heater/1 -> Sum/2
  Bus Selector/2 -> Sum1/2  "<QT>"

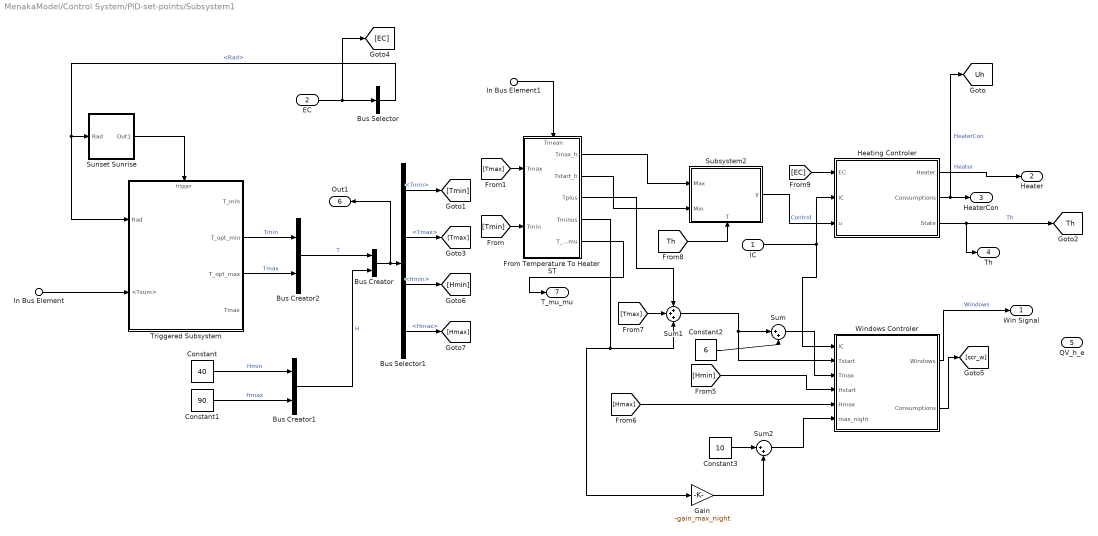
== system MenakaModel/Control System/PID-set-points/Subsystem1 ==
  IC : Inport
  EC : Inport  Port=2
  In Bus Element : Inport  Port=3  PortName=Crop  Element=Tsum
  In Bus Element1 : Inport  Port=3  PortName=Crop  Element=HeatVars.TvegMean
  Bus Creator : BusCreator  Inputs=2
  Bus Creator1 : BusCreator  Inputs=2
  Bus Creator2 : BusCreator  Inputs=2
  Bus Selector : BusSelector  OutputSignals=Rad
  Bus Selector1 : BusSelector  OutputSignals=T.Tmin,T.Tmax,H.Hmin,H.Hmax
  Constant : Constant  Value=40
  Constant1 : Constant  Value=90
  Constant2 : Constant  Value=6
  Constant3 : Constant  Value=10
  From Temperature To Heater ST : Subsystem
      settings: PortSchema="{\"entries\":[{\"content\":{\"sides\":[{\"content\":{\"connectorIds\":[\"In1\",\"In2\"]},\"type\":\"ConnectorPlacement.EquallySpacedRectSide\",\"uuid\":\"89e621f6-ef56-4bf6-8223-627da8dff273\"},{\"content\":{\"connectorIds\":[\"Out1\",\"Out2\",\"Out3\",\"Out4\",\"Out5\"],\"side\":\"RIGHT\"},\"type\":\"ConnectorPlacement.EquallySpacedRectSide\",\"uuid\":\"65a656ef-c181-4216-a438-20c957365b5a\"},{\"content\":{\"connectorIds\":[\"In3\"],\"side\":\"TOP\"},\"type\":\"ConnectorPlacement.EquallySpacedRectSide\",\"uuid\":\"92fb86b4-e089-4bcc-a83f-ddbdae4e02ae\"}]},\"type\":\"ConnectorPlacement.EquallySpacedConnector\",\"uuid\":\"5ba309fb-c1b1-411e-b7b8-8afa0be10efe\"}],\"packageUris\":[\"http://schema.mathworks.com/mf0/Connector/R2020b\"],\"version\":\"1.0\"}"
  Gain : Gain  Gain=-gain_max_night
  Heating Controler : Subsystem  AncestorBlock=HORTISIM/Climate/Controls/Heating Controler  mask{T=288, power=1000e3, A_e=6e-4, A_i=6e-4, c=1e-8}
      mask DialogControl InitialCondition Prompt: Initial Condition
      mask DialogControl Parameters Prompt: Parameters
      mask Display: image('$imagefile'); % Use "Edit Image" on toolstrip to change.
  Subsystem2 : Subsystem
      settings: PortSchema="{\"entries\":[{\"content\":{\"sides\":[{\"content\":{\"connectorIds\":[\"In1\",\"In2\"]},\"type\":\"ConnectorPlacement.EquallySpacedRectSide\",\"uuid\":\"76a0539e-cd8b-47df-82d9-61971d3be914\"},{\"content\":{\"connectorIds\":[\"Out1\"],\"side\":\"RIGHT\"},\"type\":\"ConnectorPlacement.EquallySpacedRectSide\",\"uuid\":\"93f2ebb7-6ab4-4fcc-bc7a-3583f1db6e8e\"},{\"content\":{\"connectorIds\":[],\"side\":\"TOP\"},\"type\":\"ConnectorPlacement.EquallySpacedRectSide\",\"uuid\":\"b50a0ff6-3876-4dcb-8bb9-79340929aa80\"},{\"content\":{\"connectorIds\":[\"In3\"],\"side\":\"BOTTOM\"},\"type\":\"ConnectorPlacement.EquallySpacedRectSide\",\"uuid\":\"63f2a7a5-83ef-48e2-af90-7d61b47411e6\"}]},\"type\":\"ConnectorPlacement.EquallySpacedConnector\",\"uuid\":\"d97900b9-3143-4b55-b66d-f73dd0302926\"}],\"packageUris\":[\"http://schema.mathworks.com/mf0/Connector/R2020b\"],\"version\":\"1.0\"}"
  Sum : Sum  Inputs=|++
  Sum1 : Sum  Inputs=+++
  Sum2 : Sum  Inputs=|++
  Sunset Sunrise : Subsystem
  Triggered Subsystem : Subsystem  TreatAsAtomicUnit=on
  Windows Controler : Subsystem  AncestorBlock=HORTISIM/Climate/Controls/Windows Controler  mask{Power=100, max_night=10, tau=tau_win, RadThreshold=100, AR=10}
      mask Display: image('$imagefile'); % Use "Edit Image" on toolstrip to change.
  Win Signal : Outport
  Heater : Outport  Port=2
  HeaterCon : Outport  Port=3
  Th : Outport  Port=4
  QV_h_e : Outport  Port=5
  Out1 : Outport  Port=6
  T_mu_mu : Outport  Port=7
  tag scope: Th=global, Uh=global
  wires:
  Bus Selector/1 -> Triggered Subsystem/1(Rad), Sunset Sunrise/1(Rad)  "<Rad>"
  From Temperature To Heater ST/1(Tmax_h) -> Subsystem2/1(Max)
  Bus Creator2/1 -> Bus Creator/1  "T"
  Sunset Sunrise/1(Out1) -> Triggered Subsystem/Trigger
  Sum/1 -> Windows Controler/3(Tmax)
  EC/1 -> [EC], Bus Selector/1
  Bus Selector1/4 -> [Hmax]  "<Hmax>"
  Constant1/1 -> Bus Creator1/2  "Hmax"
  Triggered Subsystem/2(T_opt_min) -> Bus Creator2/1  "Tmin"
  Bus Selector1/3 -> [Hmin]  "<Hmin>"
  IC/1 -> Heating Controler/2(IC), Windows Controler/1(IC)
  Bus Creator/1 -> Out1/1, Bus Selector1/1
  Windows Controler/1(Windows) -> Win Signal/1  "Windows"
  [Tmin] -> From Temperature To Heater ST/2(Tmin)
  In Bus Element/1 -> Triggered Subsystem/2(<Tsum>)
  Heating Controler/1(Heater) -> Heater/1  "Heater"
  Constant2/1 -> Sum/2
  [Tmax] -> From Temperature To Heater ST/1(Tmax)
  Heating Controler/2(Consumptions) -> HeaterCon/1, [Uh]  "HeaterCon"
  Triggered Subsystem/3(T_opt_max) -> Bus Creator2/2  "Tmax"
  Constant/1 -> Bus Creator1/1  "Hmin"
  Bus Selector1/1 -> [Tmin]  "<Tmin>"
  Heating Controler/3(State) -> Th/1, [Th]  "Th"
  [Hmax] -> Windows Controler/5(Hmax)
  [EC] -> Heating Controler/1(EC)
  [Hmin] -> Windows Controler/4(Hstart)
  Subsystem2/1(y) -> Heating Controler/3(u)  "Control"
  [Th] -> Subsystem2/3(T)
  Windows Controler/2(Consumptions) -> [scr_w]
  Sum1/1 -> Sum/1, Windows Controler/2(Tstart)
  Bus Creator1/1 -> Bus Creator/2  "H"
  Bus Selector1/2 -> [Tmax]  "<Tmax>"
  From Temperature To Heater ST/2(Tstart_h) -> Subsystem2/2(" Min")
  In Bus Element1/1 -> From Temperature To Heater ST/3(Tmean)
  [Tmax] -> Sum1/2
  From Temperature To Heater ST/3(Tplus) -> Sum1/1
  From Temperature To Heater ST/4(Tminus) -> Sum1/3, Gain/1
  Constant3/1 -> Sum2/1
  Sum2/1 -> Windows Controler/6(max_night)
  Gain/1 -> Sum2/2
  From Temperature To Heater ST/5(T_mu_mu) -> T_mu_mu/1

== system MenakaModel/Control System/Setpoints Control - ON//OFF/Subsystem ==
  Heater : Inport
  C1 : Inport  Port=2
  C2 : Inport  Port=3
  Bus Selector : BusSelector  OutputSignals=HeatVars.QV,HeatVars.QT,A_v,CC
  Bus Selector1 : BusSelector  OutputSignals=HeatVars.QV,HeatVars.QT,CC
  "Scalar2Bus " : Subsystem
  Sum : Sum  Inputs=+++
  Sum1 : Sum  Inputs=++|
  Sum2 : Sum  Inputs=++|
  CoCl : Outport
  wires:
  C1/1 -> Bus Selector/1
  C2/1 -> Bus Selector1/1
  Bus Selector/4 -> Sum2/2  "<CC>"
  Sum/1 -> "Scalar2Bus "/1(QV)
  Sum1/1 -> "Scalar2Bus "/2(QT)
  Bus Selector/1 -> Sum/3  "<QV>"
  Bus Selector1/1 -> Sum/1  "<QV>"
  Bus Selector1/2 -> Sum1/1  "<QT>"
  Bus Selector/3 -> "Scalar2Bus "/3(A)  "<A_v>"
  "Scalar2Bus "/1(CoCl) -> CoCl/1
  Sum2/1 -> "Scalar2Bus "/4(CC)
  Bus Selector1/3 -> Sum2/1  "<CC>"
  Heater/1 -> Sum/2
  Bus Selector/2 -> Sum1/2  "<QT>"

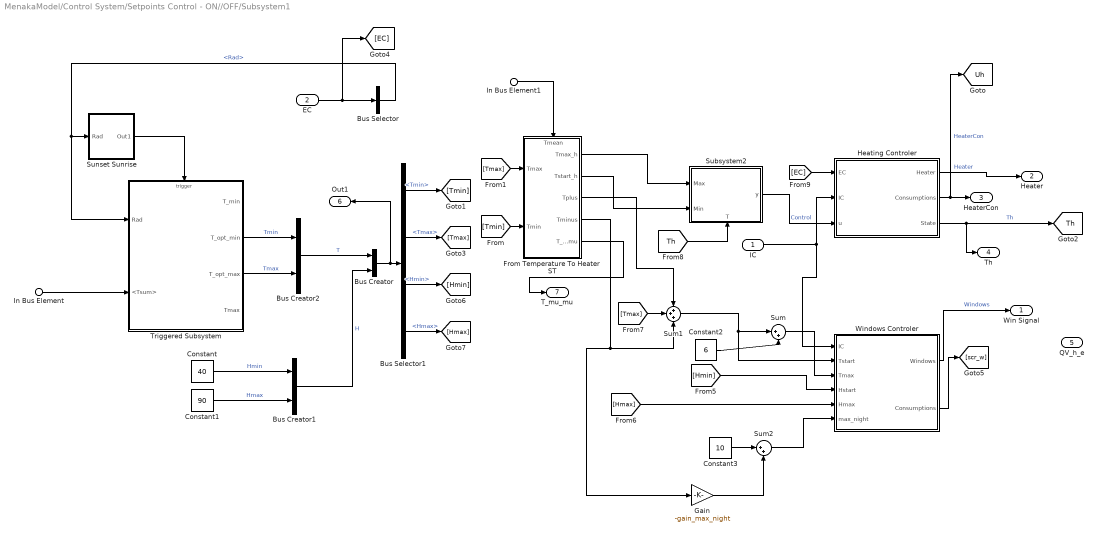
== system MenakaModel/Control System/Setpoints Control - ON//OFF/Subsystem1 ==
  IC : Inport
  EC : Inport  Port=2
  In Bus Element : Inport  Port=3  PortName=Crop  Element=Tsum
  In Bus Element1 : Inport  Port=3  PortName=Crop  Element=HeatVars.TvegMean
  Bus Creator : BusCreator  Inputs=2
  Bus Creator1 : BusCreator  Inputs=2
  Bus Creator2 : BusCreator  Inputs=2
  Bus Selector : BusSelector  OutputSignals=Rad
  Bus Selector1 : BusSelector  OutputSignals=T.Tmin,T.Tmax,H.Hmin,H.Hmax
  Constant : Constant  Value=40
  Constant1 : Constant  Value=90
  Constant2 : Constant  Value=6
  Constant3 : Constant  Value=10
  From Temperature To Heater ST : Subsystem
      settings: PortSchema="{\"entries\":[{\"content\":{\"sides\":[{\"content\":{\"connectorIds\":[\"In1\",\"In2\"]},\"type\":\"ConnectorPlacement.EquallySpacedRectSide\",\"uuid\":\"89e621f6-ef56-4bf6-8223-627da8dff273\"},{\"content\":{\"connectorIds\":[\"Out1\",\"Out2\",\"Out3\",\"Out4\",\"Out5\"],\"side\":\"RIGHT\"},\"type\":\"ConnectorPlacement.EquallySpacedRectSide\",\"uuid\":\"65a656ef-c181-4216-a438-20c957365b5a\"},{\"content\":{\"connectorIds\":[\"In3\"],\"side\":\"TOP\"},\"type\":\"ConnectorPlacement.EquallySpacedRectSide\",\"uuid\":\"92fb86b4-e089-4bcc-a83f-ddbdae4e02ae\"}]},\"type\":\"ConnectorPlacement.EquallySpacedConnector\",\"uuid\":\"5ba309fb-c1b1-411e-b7b8-8afa0be10efe\"}],\"packageUris\":[\"http://schema.mathworks.com/mf0/Connector/R2020b\"],\"version\":\"1.0\"}"
  Gain : Gain  Gain=-gain_max_night
  Heating Controler : Subsystem  AncestorBlock=HORTISIM/Climate/Controls/Heating Controler  mask{T=288, power=1000e3, A_e=6e-4, A_i=6e-4, c=1e-8}
      mask DialogControl InitialCondition Prompt: Initial Condition
      mask DialogControl Parameters Prompt: Parameters
      mask Display: image('$imagefile'); % Use "Edit Image" on toolstrip to change.
  Subsystem2 : Subsystem
      settings: PortSchema="{\"entries\":[{\"content\":{\"sides\":[{\"content\":{\"connectorIds\":[\"In1\",\"In2\"]},\"type\":\"ConnectorPlacement.EquallySpacedRectSide\",\"uuid\":\"76a0539e-cd8b-47df-82d9-61971d3be914\"},{\"content\":{\"connectorIds\":[\"Out1\"],\"side\":\"RIGHT\"},\"type\":\"ConnectorPlacement.EquallySpacedRectSide\",\"uuid\":\"93f2ebb7-6ab4-4fcc-bc7a-3583f1db6e8e\"},{\"content\":{\"connectorIds\":[],\"side\":\"TOP\"},\"type\":\"ConnectorPlacement.EquallySpacedRectSide\",\"uuid\":\"b50a0ff6-3876-4dcb-8bb9-79340929aa80\"},{\"content\":{\"connectorIds\":[\"In3\"],\"side\":\"BOTTOM\"},\"type\":\"ConnectorPlacement.EquallySpacedRectSide\",\"uuid\":\"63f2a7a5-83ef-48e2-af90-7d61b47411e6\"}]},\"type\":\"ConnectorPlacement.EquallySpacedConnector\",\"uuid\":\"d97900b9-3143-4b55-b66d-f73dd0302926\"}],\"packageUris\":[\"http://schema.mathworks.com/mf0/Connector/R2020b\"],\"version\":\"1.0\"}"
  Sum : Sum  Inputs=|++
  Sum1 : Sum  Inputs=+++
  Sum2 : Sum  Inputs=|++
  Sunset Sunrise : Subsystem
  Triggered Subsystem : Subsystem  TreatAsAtomicUnit=on
  Windows Controler : Subsystem  AncestorBlock=HORTISIM/Climate/Controls/Windows Controler  mask{Power=100, max_night=10, tau=tau_win, RadThreshold=100, AR=10}
      mask Display: image('$imagefile'); % Use "Edit Image" on toolstrip to change.
  Win Signal : Outport
  Heater : Outport  Port=2
  HeaterCon : Outport  Port=3
  Th : Outport  Port=4
  QV_h_e : Outport  Port=5
  Out1 : Outport  Port=6
  T_mu_mu : Outport  Port=7
  tag scope: Th=global, Uh=global
  wires:
  Bus Selector/1 -> Triggered Subsystem/1(Rad), Sunset Sunrise/1(Rad)  "<Rad>"
  From Temperature To Heater ST/1(Tmax_h) -> Subsystem2/1(Max)
  Bus Creator2/1 -> Bus Creator/1  "T"
  Sunset Sunrise/1(Out1) -> Triggered Subsystem/Trigger
  Sum/1 -> Windows Controler/3(Tmax)
  EC/1 -> [EC], Bus Selector/1
  Bus Selector1/4 -> [Hmax]  "<Hmax>"
  Constant1/1 -> Bus Creator1/2  "Hmax"
  Triggered Subsystem/2(T_opt_min) -> Bus Creator2/1  "Tmin"
  Bus Selector1/3 -> [Hmin]  "<Hmin>"
  IC/1 -> Heating Controler/2(IC), Windows Controler/1(IC)
  Bus Creator/1 -> Out1/1, Bus Selector1/1
  Windows Controler/1(Windows) -> Win Signal/1  "Windows"
  [Tmin] -> From Temperature To Heater ST/2(Tmin)
  In Bus Element/1 -> Triggered Subsystem/2(<Tsum>)
  Heating Controler/1(Heater) -> Heater/1  "Heater"
  Constant2/1 -> Sum/2
  [Tmax] -> From Temperature To Heater ST/1(Tmax)
  Heating Controler/2(Consumptions) -> HeaterCon/1, [Uh]  "HeaterCon"
  Triggered Subsystem/3(T_opt_max) -> Bus Creator2/2  "Tmax"
  Constant/1 -> Bus Creator1/1  "Hmin"
  Bus Selector1/1 -> [Tmin]  "<Tmin>"
  Heating Controler/3(State) -> Th/1, [Th]  "Th"
  [Hmax] -> Windows Controler/5(Hmax)
  [EC] -> Heating Controler/1(EC)
  [Hmin] -> Windows Controler/4(Hstart)
  Subsystem2/1(y) -> Heating Controler/3(u)  "Control"
  [Th] -> Subsystem2/3(T)
  Windows Controler/2(Consumptions) -> [scr_w]
  Sum1/1 -> Sum/1, Windows Controler/2(Tstart)
  Bus Creator1/1 -> Bus Creator/2  "H"
  Bus Selector1/2 -> [Tmax]  "<Tmax>"
  From Temperature To Heater ST/2(Tstart_h) -> Subsystem2/2(" Min")
  In Bus Element1/1 -> From Temperature To Heater ST/3(Tmean)
  [Tmax] -> Sum1/2
  From Temperature To Heater ST/3(Tplus) -> Sum1/1
  From Temperature To Heater ST/4(Tminus) -> Sum1/3, Gain/1
  Constant3/1 -> Sum2/1
  Sum2/1 -> Windows Controler/6(max_night)
  Gain/1 -> Sum2/2
  From Temperature To Heater ST/5(T_mu_mu) -> T_mu_mu/1

== system MenakaModel/Subsystem1/For Each Subsystem/Subsystem ==
  I1 : Inport
  I2 : Inport  Port=2
  Abs : Abs  ZeroCross=off  SaturateOnIntegerOverflow=off
  If : If  IfExpression=u1 < 1e-9  ZeroCross=off
  If Action Subsystem : Subsystem  TreatAsAtomicUnit=on
  If Action Subsystem1 : Subsystem  TreatAsAtomicUnit=on
  Merge : Merge
  Merge1 : Merge
  Sum : Sum  Inputs=|++
  f1 : Outport
  f2 : Outport  Port=2
  fT : Outport  Port=3
  wires:
  I1/1 -> If Action Subsystem1/1(In1), Sum/1
  I2/1 -> If Action Subsystem1/2(In2), Sum/2
  Sum/1 -> fT/1, [T]
  If/1 -> If Action Subsystem/Action
  If/2 -> If Action Subsystem1/Action
  [T] -> If Action Subsystem1/3(In3)
  If Action Subsystem/2(Out2) -> Merge/1
  If Action Subsystem1/2(Out2) -> Merge/2
  Merge/1 -> f2/1
  Merge1/1 -> f1/1
  If Action Subsystem1/1(Out1) -> Merge1/2
  If Action Subsystem/1(Out1) -> Merge1/1
  Abs/1 -> If/1
  [T] -> Abs/1

== system MenakaModel/Subsystem1/Subsystem/If Action Subsystem ==
  Action Port : ActionPort  ActionPortLabel=if(u1 < 1e-9)
  Constant : Constant  Value=0
  Constant1 : Constant  Value=0
  Out1 : Outport
  Out2 : Outport  Port=2
  wires:
  Constant/1 -> Out1/1
  Constant1/1 -> Out2/1

== system MenakaModel/Subsystem1/Subsystem/If Action Subsystem1 ==
  In1 : Inport
  In2 : Inport  Port=2
  In3 : Inport  Port=3
  Action Port : ActionPort  ActionPortLabel=else
  Divide : Product  Inputs=*/
  Divide1 : Product  Inputs=*/
  Out1 : Outport
  Out2 : Outport  Port=2
  wires:
  In1/1 -> Divide/1
  In2/1 -> Divide1/1
  In3/1 -> Divide1/2, Divide/2
  Divide/1 -> Out1/1
  Divide1/1 -> Out2/1

== system MenakaModel/Control System/Control System Proportional (Ti) + Tmu /Heating Controler/Subsystem ==
  T_i : Inport
  Q_h : Inport  Port=2
  T_e : Inport  Port=3
  Th : Inport  Port=4
  Constant : Constant  Value=A_i
  Constant1 : Constant  Value=c
  Constant2 : Constant  Value=A_e
  Product : Product
  Subsystem1 : Subsystem
  Subsystem2 : Subsystem
  Sum : Sum  Inputs=|-+-
  QV_h_i : Outport
  dT_h_dt : Outport  Port=2
  QV_h_e : Outport  Port=3
  wires:
  T_i/1 -> Subsystem1/1(Ti)
  Constant/1 -> Subsystem1/2(A_h_exp)
  Th/1 -> Subsystem2/3(Th), Subsystem1/3(Th)
  T_e/1 -> Subsystem2/1(Te)
  Subsystem1/1(QV_h_i) -> QV_h_i/1, Sum/1
  Subsystem2/1(QV_h_e) -> QV_h_e/1, Sum/3
  Q_h/1 -> Sum/2
  Sum/1 -> Product/1
  Constant1/1 -> Product/2
  Product/1 -> dT_h_dt/1
  Constant2/1 -> Subsystem2/2(A_h_exp)

== system MenakaModel/Control System/Control System Proportional (Ti) + Tmu /Heating Controler/Subsystem2 ==
  " Min" : Inport
  Max : Inport  Port=2
  T : Inport  Port=3
  Divide : Product  Inputs=*/
  Gain : Gain  Gain=0.5
  Gain1 : Gain  Gain=0.5
  Minus : Sum  Inputs=+-
  Minus1 : Sum  Inputs=+-
  Saturation : Saturate  UpperLimit=1  LowerLimit=0
  Sum : Sum  Inputs=|++
  y : Outport
  wires:
  Saturation/1 -> y/1
  Max/1 -> Gain1/1
  T/1 -> Minus/1
  Minus1/1 -> Divide/2
  Minus/1 -> Divide/1
  Divide/1 -> Saturation/1
  " Min"/1 -> Gain/1, Minus1/1
  Gain/1 -> Sum/1
  Gain1/1 -> Sum/2
  Sum/1 -> [Tmu]
  [Tmu] -> Minus1/2, Minus/2

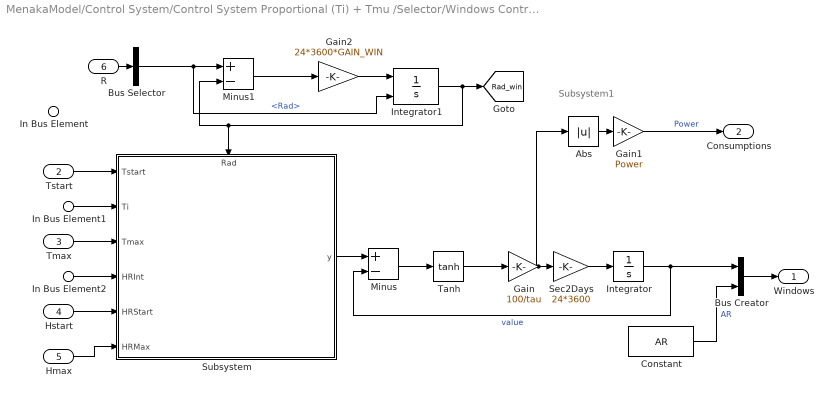
== system MenakaModel/Control System/Control System Proportional (Ti) + Tmu /Selector/Windows Controler ==
  note: Subsystem1
  In Bus Element : Inport  PortName=IC  Element=QS.R_int
  In Bus Element1 : Inport  PortName=IC  Element=Temp.Tair
  In Bus Element2 : Inport  PortName=IC  Element=Gas.HRInt
  Tstart : Inport  Port=2
  Tmax : Inport  Port=3
  Hstart : Inport  Port=4
  Hmax : Inport  Port=5
  R : Inport  Port=6
  Abs : Abs  ZeroCross=off  SaturateOnIntegerOverflow=off
  Bus Creator : BusCreator  Inputs=2
  Bus Selector : BusSelector  OutputSignals=Rad
  Constant : Constant  Value=AR
  Gain : Gain  Gain=100/tau
  Gain1 : Gain  Gain=Power
  Gain2 : Gain  Gain=24*3600*GAIN_WIN
  Integrator : Integrator
  Integrator1 : Integrator  InitialConditionSource=external
  Minus : Sum  Inputs=+-
  Minus1 : Sum  Inputs=+-
  Sec2Days : Gain  Gain=24*3600
  Subsystem : Subsystem
      settings: PortSchema="{\"entries\":[{\"content\":{\"sides\":[{\"content\":{\"connectorIds\":[\"In1\",\"In2\",\"In3\",\"In4\",\"In5\",\"In6\"]},\"type\":\"ConnectorPlacement.EquallySpacedRectSide\",\"uuid\":\"18d05740-181f-409c-94ea-b42b6e57ea74\"},{\"content\":{\"connectorIds\":[\"Out1\"],\"side\":\"RIGHT\"},\"type\":\"ConnectorPlacement.EquallySpacedRectSide\",\"uuid\":\"978406c3-d241-44cd-a3e7-fe734e3a171e\"},{\"content\":{\"connectorIds\":[\"In7\"],\"side\":\"TOP\"},\"type\":\"ConnectorPlacement.EquallySpacedRectSide\",\"uuid\":\"b3c10a0e-c6d9-4444-97f2-9f0c7dea8ec9\"}]},\"type\":\"ConnectorPlacement.EquallySpacedConnector\",\"uuid\":\"429bf3f5-5806-495e-b66b-96810540e6d1\"}],\"packageUris\":[\"http://schema.mathworks.com/mf0/Connector/R2020b\"],\"version\":\"1.0\"}"
  Tanh : Trigonometry  Operator=tanh
  Windows : Outport
  Consumptions : Outport  Port=2
  tag scope: Rad_win=global
  wires:
  Tstart/1 -> Subsystem/1(Tstart)
  In Bus Element1/1 -> Subsystem/2(Ti)
  Tmax/1 -> Subsystem/3(Tmax)
  Integrator/1 -> Bus Creator/1, Minus/2  "value"
  In Bus Element2/1 -> Subsystem/4(HRInt)
  Hstart/1 -> Subsystem/5(HRStart)
  Hmax/1 -> Subsystem/6(HRMax)
  Subsystem/1(y) -> Minus/1
  Sec2Days/1 -> Integrator/1
  Gain1/1 -> Consumptions/1  "Power"
  Abs/1 -> Gain1/1
  Gain/1 -> Abs/1, Sec2Days/1
  Tanh/1 -> Gain/1
  Minus/1 -> Tanh/1
  Bus Creator/1 -> Windows/1
  Constant/1 -> Bus Creator/2  "AR"
  Gain2/1 -> Integrator1/1
  Minus1/1 -> Gain2/1
  Integrator1/1 -> [Rad_win], Subsystem/7(Rad), Minus1/2
  R/1 -> Bus Selector/1
  Bus Selector/1 -> Integrator1/2, Minus1/1  "<Rad>"

== system MenakaModel/Control System/Control System Proportional (Ti) + Tmu /Subsystem/Scalar2Bus  ==
  QV : Inport
  QT : Inport  Port=2
  A : Inport  Port=3
  CC : Inport  Port=4
  Bus Creator : BusCreator  Inputs=4
  CoCl : Outport
  wires:
  A/1 -> Bus Creator/3  "A"
  CC/1 -> Bus Creator/4  "CC"
  QV/1 -> Bus Creator/1  "QV"
  Bus Creator/1 -> CoCl/1
  QT/1 -> Bus Creator/2  "QT"

== system MenakaModel/Control System/Control System Proportional (Ti) + Tmu Windows Relay/Heating Controler/Subsystem ==
  T_i : Inport
  Q_h : Inport  Port=2
  T_e : Inport  Port=3
  Th : Inport  Port=4
  Constant : Constant  Value=A_i
  Constant1 : Constant  Value=c
  Constant2 : Constant  Value=A_e
  Product : Product
  Subsystem1 : Subsystem
  Subsystem2 : Subsystem
  Sum : Sum  Inputs=|-+-
  QV_h_i : Outport
  dT_h_dt : Outport  Port=2
  QV_h_e : Outport  Port=3
  wires:
  T_i/1 -> Subsystem1/1(Ti)
  Constant/1 -> Subsystem1/2(A_h_exp)
  Th/1 -> Subsystem2/3(Th), Subsystem1/3(Th)
  T_e/1 -> Subsystem2/1(Te)
  Subsystem1/1(QV_h_i) -> QV_h_i/1, Sum/1
  Subsystem2/1(QV_h_e) -> QV_h_e/1, Sum/3
  Q_h/1 -> Sum/2
  Sum/1 -> Product/1
  Constant1/1 -> Product/2
  Product/1 -> dT_h_dt/1
  Constant2/1 -> Subsystem2/2(A_h_exp)
